simulink model "practica1"  (R2023a)
settings: Solver=VariableStepAuto  StartTime=0.0  StopTime=10.0  MaxStep=0.01  RelTol=1e-3
values from neighbouring files (symbols this model uses):
  g = 9.81    [practica1.m]
  l1 = .3    (= 0.3)    [practica1.m]
  l2 = .25    (= 0.25)    [practica1.m]
  m1 = .2    (= 0.2)    [practica1.m]
  m2 = .1    (= 0.1)    [practica1.m]
settings Model: Creator=Pablo  LastModifiedBy=Pablo

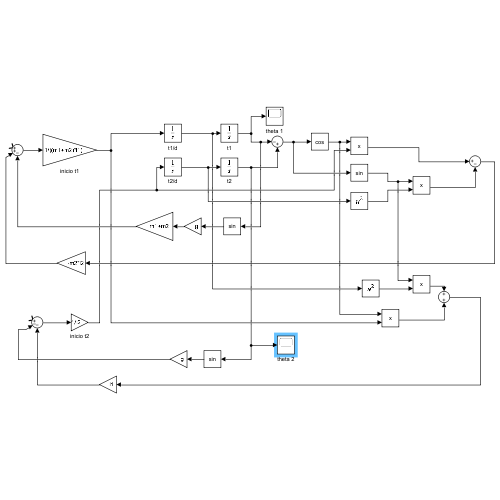
[thumbnail: Simulink's stored preview of the top-level diagram]
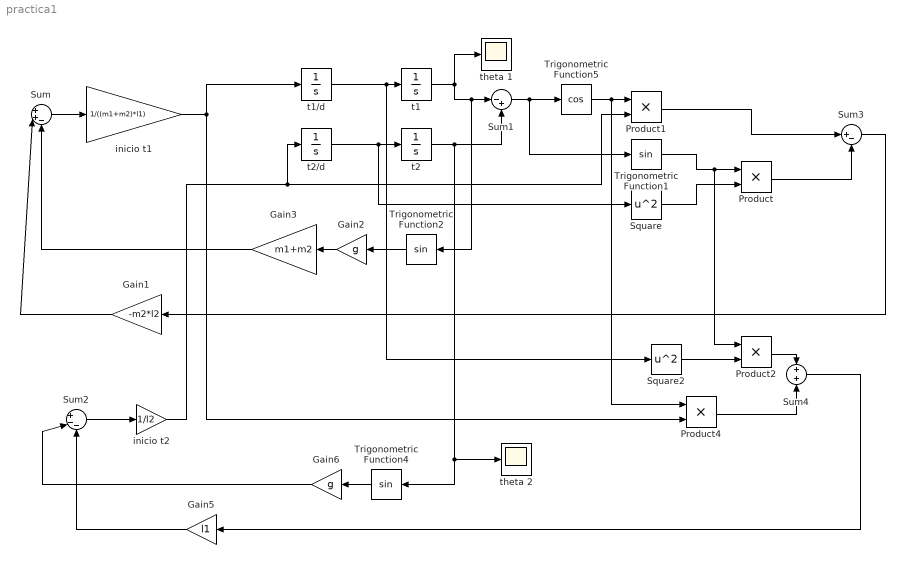
== system practica1 ==
  Gain1 : Gain  Gain=-m2*l2
  Gain2 : Gain  Gain=g
  Gain3 : Gain  Gain=m1+m2
  Gain5 : Gain  Gain=l1
  Gain6 : Gain  Gain=g
  Product{,1..2,4} (4 alike) : Product
  Square : Math  Operator=square
  Square2 : Math  Operator=square
  Sum : Sum  Inputs=|++-
  Sum1 : Sum  Inputs=|-+
  Sum2 : Sum  Inputs=|+--
  Sum3 : Sum  Inputs=|+-
  Sum4 : Sum
  Trigonometric Function1 : Trigonometry
  Trigonometric Function2 : Trigonometry
  Trigonometric Function4 : Trigonometry
  Trigonometric Function5 : Trigonometry  Operator=cos
  inicio t1 : Gain  Gain=1/((m1+m2)*l1)
  inicio t2 : Gain  Gain=1/l2
  t1 : Integrator
  t1/d : Integrator
  t2 : Integrator  InitialCondition=(35*pi)/180
  t2/d : Integrator
  theta 1 : Scope
  theta 2 : Scope
  wires:
  inicio t2/1 -> t2/d/1, Product1/2
  t2/d/1 -> Square/1, t2/1
  t1/d/1 -> Square2/1, t1/1
  Gain1/1 -> Sum/2
  t2/1 -> Sum1/2, Trigonometric Function4/1, theta 2/1
  t1/1 -> Trigonometric Function2/1, Sum1/1, theta 1/1
  Gain5/1 -> Sum2/3
  Sum/1 -> inicio t1/1
  Sum2/1 -> inicio t2/1
  Gain2/1 -> Gain3/1
  Trigonometric Function2/1 -> Gain2/1
  Gain3/1 -> Sum/3
  Trigonometric Function4/1 -> Gain6/1
  Gain6/1 -> Sum2/2
  Sum3/1 -> Gain1/1
  Product/1 -> Sum3/2
  Trigonometric Function1/1 -> Product2/1, Product/1
  Square/1 -> Product/2
  Product1/1 -> Sum3/1
  Sum1/1 -> Trigonometric Function1/1, Trigonometric Function5/1
  Trigonometric Function5/1 -> Product4/1, Product1/1
  inicio t1/1 -> Product4/2, t1/d/1
  Product4/1 -> Sum4/2
  Sum4/1 -> Gain5/1
  Square2/1 -> Product2/2
  Product2/1 -> Sum4/1
